simulink model "sampleModel1666_3_sub"  (R2023a)
settings: Solver=VariableStepAuto  StartTime=0.0  StopTime=10.0  RelTol=1e-3
libraries: hdlsllib x5, simulink x2
settings Model: Creator=user1  LastModifiedBy=user1
settings OptimizationCC: BlockReduction=off  ConditionallyExecuteInputs=off

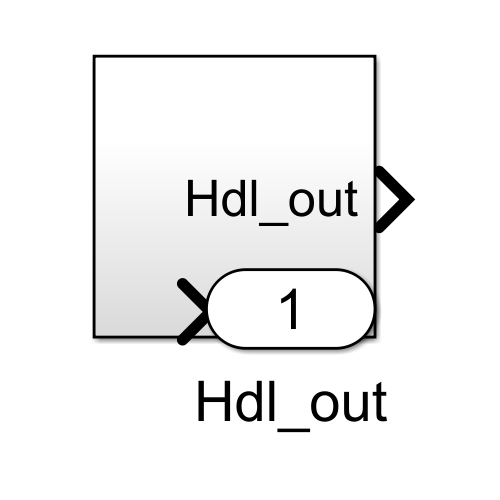
[thumbnail: Simulink's stored preview of the top-level diagram]
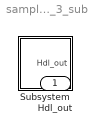
== system sampleModel1666_3_sub ==
  Subsystem : Subsystem
  Hdl_out : Outport  OutDataTypeStr=uint8

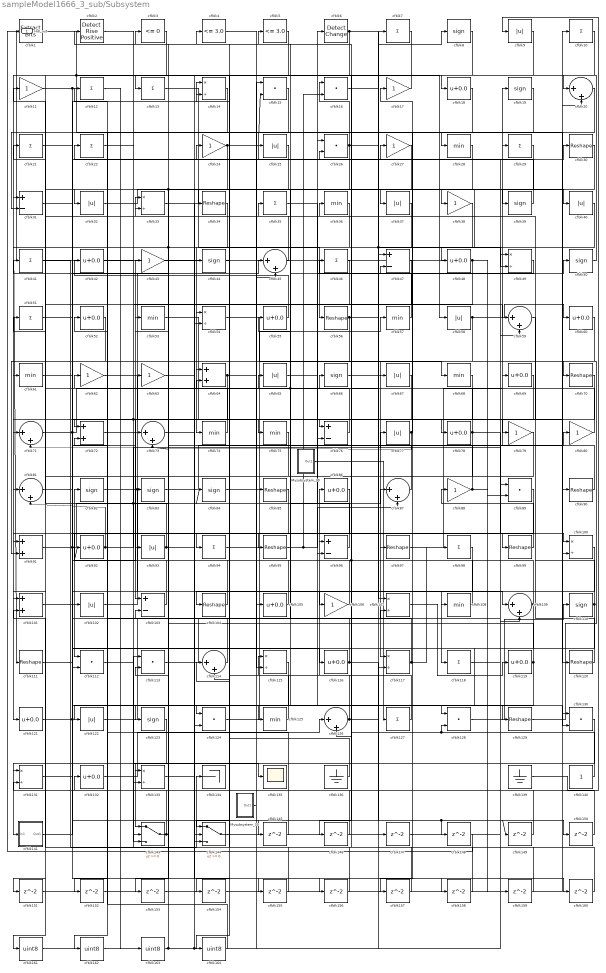
== system sampleModel1666_3_sub/Subsystem ==
  Mysubsystem_30 : Subsystem  TreatAsAtomicUnit=on  RTWFcnName=Mysubsystem_30
      settings: RTWFcnNameOpts=User specified  RTWFileNameOpts=Use function name
  Mysubsystem_33 : Subsystem  TreatAsAtomicUnit=on  RTWFcnName=Mysubsystem_33
      settings: RTWFcnNameOpts=User specified  RTWFileNameOpts=Use function name
  cfblk1 : simulink/Logic and Bit Operations/Extract Bits  bitsToExtract=Upper half  numBits=8  bitIdxRange=[0 7]  outScalingMode=Preserve fixed-point scaling
      settings: LibrarySourceBlock=|
      | hdlsllib/Logic and Bit
      | Operations/Extract Bits
  cfblk{7,10,12..13,21..22,29,35,41,46,51,94,98,118,127} (15 alike) : Sum  Inputs=+  OutDataTypeStr=uint8
  cfblk{14,33,49,54,100,107,115,117,131,133} (10 alike) : Product  Inputs=*/  OutDataTypeStr=uint8  RndMeth=Zero  SaturateOnIntegerOverflow=on
  cfblk{64,72,91,101} (4 alike) : Sum  OutDataTypeStr=uint8
  cfblk{9,25,32,37,40,58,65,67,77,93,102,122} (12 alike) : Abs  OutDataTypeStr=uint8  SaturateOnIntegerOverflow=off
  cfblk{31,47,76,96,103} (5 alike) : Sum  Inputs=+-  OutDataTypeStr=uint8
  cfblk{30,34,56,70,85,90,95,97,99,104,111,120,129} (13 alike) : Reshape
  cfblk{18,42,48,52,55,60,69,78,86,92,105,116,119,121,132} (15 alike) : Bias  Bias=0.0  SaturateOnIntegerOverflow=off
  cfblk{11,17,24,27,38,43,62..63,79..80,88,106} (12 alike) : Gain  OutDataTypeStr=uint8
  cfblk{28,36,53,57,61,68,74..75,108,125} (10 alike) : MinMax  OutDataTypeStr=uint8
  cfblk{20,45,59,71,73,81,87,109,114,126} (10 alike) : Sum  Inputs=|++  OutDataTypeStr=uint8
  cfblk{8,19,39,44,50,66,82..84,110,123} (11 alike) : Signum
  cfblk{15..16,26,89,112..113,124,128,130} (9 alike) : DotProduct  OutDataTypeStr=uint8
  cfblk134 : Terminator
  cfblk135 : Scope
  cfblk136 : Ground
  cfblk139 : Ground
  cfblk140 : Constant  OutDataTypeStr=uint8  SampleTime=-1
  cfblk141 : Subsystem
      settings: LibrarySourceBlock=|
      | hdlsllib/Ports &
      | Subsystems/Subsystem
  cfblk143 : Switch  OutDataTypeStr=uint8  SaturateOnIntegerOverflow=off  InputSameDT=off
  cfblk144 : Switch  OutDataTypeStr=uint8  SaturateOnIntegerOverflow=off  InputSameDT=off
  cfblk{145..160} (16 alike) : Delay  SampleTime=1
  cfblk{161..164} (4 alike) : DataTypeConversion  OutDataTypeStr=uint8  SaturateOnIntegerOverflow=off  RndMeth=Floor
  cfblk2 : hdlsllib/Logic and Bit Operations/Detect Rise Positive  vinit=0  OutDataTypeStr=uint8
  cfblk3 : hdlsllib/Logic and Bit Operations/Compare To Zero  relop=<=  OutDataTypeStr=uint8
  cfblk4 : hdlsllib/Logic and Bit Operations/Compare To Constant  relop=<=  const=3.0  OutDataTypeStr=uint8
  cfblk5 : hdlsllib/Logic and Bit Operations/Compare To Constant  relop=<=  const=3.0  OutDataTypeStr=uint8
  cfblk6 : simulink/Logic and Bit Operations/Detect Change  vinit=0  OutDataTypeStr=uint8
      settings: LibrarySourceBlock=|
      | hdlsllib/Logic and Bit
      | Operations/Detect
      | Change
  Hdl_out : Outport  OutDataTypeStr=uint8
  wires:
  cfblk132/1 -> cfblk126/1
  cfblk34/1 -> cfblk74/1
  cfblk143/1 -> cfblk83/1, cfblk132/1
  cfblk20/1 -> cfblk121/1
  cfblk89/1 -> cfblk112/1
  cfblk8/1 -> cfblk31/1
  cfblk1/1 -> cfblk58/1, cfblk28/1
  cfblk110/1 -> cfblk112/2, cfblk62/1
  cfblk103/1 -> cfblk82/1
  cfblk104/1 -> cfblk43/1
  cfblk57/1 -> cfblk32/1
  cfblk128/1 -> cfblk110/1
  cfblk124/1 -> cfblk57/1
  cfblk41/1 -> cfblk134/1
  cfblk81/1 -> cfblk45/1
  cfblk80/1 -> cfblk36/1
  cfblk72/1 -> cfblk27/1
  cfblk102/1 -> cfblk66/1
  cfblk42/1 -> cfblk75/1
  cfblk68/1 -> cfblk103/1
  cfblk121/1 -> cfblk107/2, cfblk149/1, cfblk148/1
  cfblk85/1 -> cfblk161/1
  cfblk129/1 -> cfblk70/1
  cfblk33/1 -> cfblk40/1
  cfblk96/1 -> cfblk65/1
  cfblk82/1 -> cfblk59/2, cfblk118/1
  cfblk123/1 -> cfblk141/1(In1)
  cfblk114/1 -> cfblk53/1
  cfblk126/1 -> cfblk8/1, cfblk86/1
  cfblk93/1 -> cfblk155/1, cfblk11/1
  cfblk86/1 -> cfblk94/1
  cfblk90/1 -> cfblk19/1
  cfblk66/1 -> cfblk117/1
  cfblk40/1 -> cfblk97/1
  cfblk18/1 -> cfblk67/1
  cfblk67/1 -> cfblk125/1
  cfblk71/1 -> cfblk100/1, cfblk7/1
  cfblk74/1 -> cfblk3/1
  cfblk56/1 -> cfblk123/1, cfblk47/1
  cfblk53/1 -> cfblk120/1
  cfblk77/1 -> cfblk71/2, cfblk17/1
  cfblk91/1 -> cfblk160/1, cfblk6/1
  cfblk5/1 -> cfblk104/1
  cfblk140/1 -> cfblk128/2, cfblk2/1, cfblk92/1
  cfblk117/1 -> cfblk98/1, cfblk52/1
  cfblk9/1 -> cfblk18/1
  cfblk94/1 -> cfblk26/1
  cfblk97/1 -> cfblk69/1
  cfblk84/1 -> cfblk105/1
  cfblk61/1 -> cfblk109/1
  cfblk12/1 -> cfblk163/1
  cfblk36/1 -> cfblk73/2, cfblk111/1
  cfblk30/1 -> cfblk91/1
  cfblk127/1 -> cfblk22/1
  cfblk26/1 -> cfblk16/1, cfblk95/1, cfblk39/1
  cfblk55/1 -> cfblk42/1
  cfblk108/1 -> cfblk96/1
  cfblk109/1 -> cfblk128/1, cfblk5/1
  cfblk133/1 -> cfblk87/1
  cfblk62/1 -> cfblk78/1
  cfblk21/1 -> cfblk102/1
  cfblk64/1 -> cfblk144/3, cfblk96/2
  cfblk69/1 -> cfblk81/1
  cfblk107/1 -> cfblk119/1
  cfblk95/1 -> cfblk16/2, cfblk87/2
  cfblk13/1 -> cfblk56/1
  cfblk125/1 -> cfblk115/1
  cfblk4/1 -> cfblk106/1
  cfblk6/1 -> cfblk64/1, cfblk49/2, cfblk99/1
  cfblk83/1 -> cfblk10/1
  cfblk32/1 -> cfblk38/1
  cfblk38/1 -> cfblk54/1
  cfblk31/1 -> cfblk116/1
  cfblk50/1 -> cfblk20/1
  cfblk88/1 -> cfblk159/1, cfblk41/1
  cfblk99/1 -> cfblk88/1
  cfblk49/1 -> cfblk47/2
  cfblk130/1 -> cfblk143/1
  cfblk52/1 -> cfblk61/1
  cfblk11/1 -> cfblk76/1, cfblk90/1
  cfblk100/1 -> cfblk144/1
  cfblk15/1 -> cfblk72/1
  cfblk131/1 -> cfblk14/1
  cfblk16/1 -> cfblk107/1
  cfblk43/1 -> cfblk144/2
  cfblk27/1 -> cfblk37/1
  cfblk106/1 -> cfblk33/1
  cfblk46/1 -> cfblk71/1
  cfblk113/1 -> cfblk30/1
  cfblk54/1 -> cfblk68/1
  cfblk24/1 -> cfblk124/2, cfblk15/2
  cfblk28/1 -> cfblk115/2
  cfblk105/1 -> cfblk4/1
  cfblk47/1 -> cfblk133/1
  cfblk17/1 -> cfblk13/1
  cfblk75/1 -> cfblk133/2
  cfblk65/1 -> cfblk50/1
  cfblk101/1 -> cfblk130/2
  cfblk118/1 -> cfblk80/1
  cfblk51/1 -> cfblk29/1
  cfblk58/1 -> cfblk143/3, cfblk60/1
  cfblk78/1 -> cfblk100/2, cfblk131/1, cfblk46/1
  cfblk39/1 -> cfblk24/1
  cfblk120/1 -> cfblk33/2
  cfblk116/1 -> cfblk150/1, cfblk55/1
  cfblk48/1 -> Hdl_out/1, cfblk154/1, cfblk89/2
  cfblk45/1 -> cfblk21/1
  cfblk111/1 -> cfblk93/1
  cfblk122/1 -> cfblk34/1
  cfblk98/1 -> cfblk108/1
  cfblk59/1 -> cfblk79/1
  cfblk37/1 -> cfblk114/2
  cfblk115/1 -> cfblk122/1
  cfblk22/1 -> cfblk59/1
  cfblk144/1 -> cfblk89/1
  cfblk25/1 -> cfblk153/1, cfblk152/1
  cfblk60/1 -> cfblk91/2
  cfblk136/1 -> cfblk14/2
  cfblk19/1 -> cfblk31/2
  cfblk87/1 -> cfblk35/1
  cfblk3/1 -> cfblk101/1
  cfblk119/1 -> cfblk63/1, cfblk124/1
  cfblk141/1(Out1) -> cfblk73/1
  cfblk139/1 -> cfblk9/1
  cfblk76/1 -> cfblk51/1, cfblk25/1
  cfblk92/1 -> cfblk81/2, cfblk84/1, cfblk77/1
  cfblk29/1 -> cfblk48/1
  cfblk2/1 -> cfblk76/2, cfblk135/1
  cfblk10/1 -> cfblk54/2
  cfblk35/1 -> cfblk129/1
  cfblk112/1 -> cfblk145/1
  cfblk145/1 -> cfblk72/2
  cfblk7/1 -> cfblk146/1
  cfblk146/1 -> cfblk114/1
  cfblk147/1 -> cfblk109/2
  cfblk148/1 -> cfblk1/1
  cfblk149/1 -> cfblk101/2
  cfblk150/1 -> cfblk126/2
  cfblk70/1 -> cfblk151/1
  cfblk151/1 -> cfblk130/1
  cfblk152/1 -> cfblk45/2
  cfblk153/1 -> cfblk117/2
  cfblk154/1 -> cfblk20/2
  cfblk155/1 -> cfblk64/2
  cfblk73/1 -> cfblk156/1
  cfblk156/1 -> cfblk113/1
  cfblk79/1 -> cfblk157/1
  cfblk157/1 -> cfblk103/2
  cfblk63/1 -> cfblk158/1
  cfblk158/1 -> cfblk26/2
  cfblk159/1 -> cfblk143/2
  cfblk160/1 -> cfblk131/2
  cfblk161/1 -> cfblk44/1, cfblk49/1
  cfblk14/1 -> cfblk162/1
  cfblk162/1 -> cfblk85/1
  cfblk163/1 -> cfblk113/2, cfblk147/1
  cfblk44/1 -> cfblk164/1
  cfblk164/1 -> cfblk12/1
  Mysubsystem_30/1(Out1) -> cfblk127/1
  Mysubsystem_33/1(Out1) -> cfblk15/1

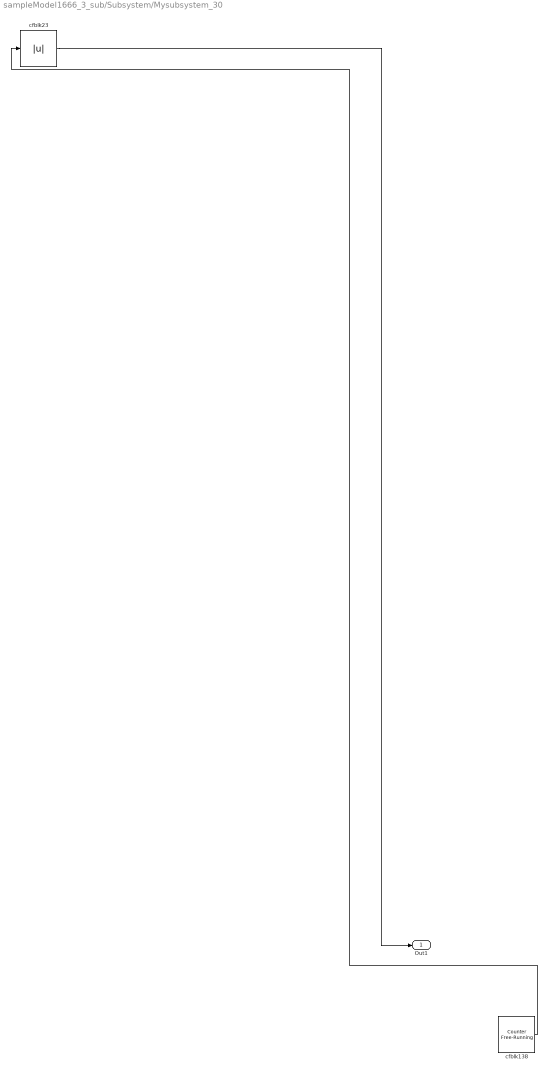
== system sampleModel1666_3_sub/Subsystem/Mysubsystem_30 ==
  cfblk138 : hdlsllib/Sources/Counter Free-Running  NumBits=16  tsamp=-1
  cfblk23 : Abs  SaturateOnIntegerOverflow=off
  Out1 : Outport
  wires:
  cfblk23/1 -> Out1/1
  cfblk138/1 -> cfblk23/1

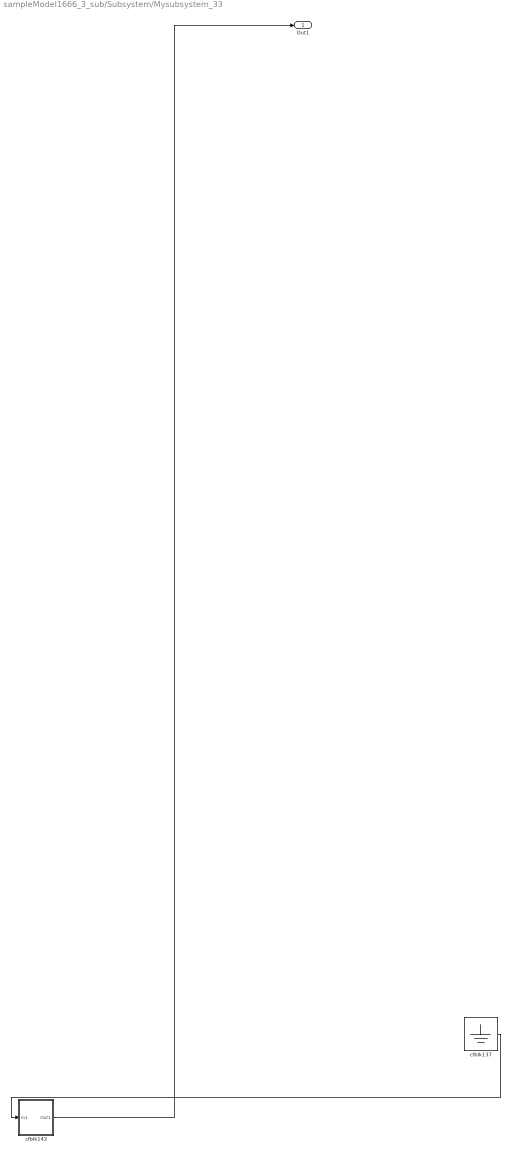
== system sampleModel1666_3_sub/Subsystem/Mysubsystem_33 ==
  cfblk137 : Ground
  cfblk142 : Subsystem
      settings: LibrarySourceBlock=|
      | hdlsllib/Ports &
      | Subsystems/Subsystem
  Out1 : Outport
  wires:
  cfblk142/1(Out1) -> Out1/1
  cfblk137/1 -> cfblk142/1(In1)

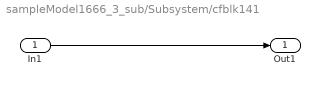
== system sampleModel1666_3_sub/Subsystem/cfblk141 ==
  In1 : Inport
  Out1 : Outport
  wires:
  In1/1 -> Out1/1

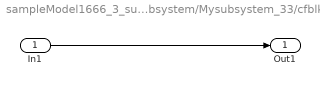
== system sampleModel1666_3_sub/Subsystem/Mysubsystem_33/cfblk142 ==
  In1 : Inport
  Out1 : Outport
  wires:
  In1/1 -> Out1/1
